simulink model "BrakeActuator"  (Simulink 7.4)
settings: Solver=ode45  StartTime=0.0  StopTime=10.0  RelTol=1e-3
undefined symbols (not defined in the file): Kf, PBmax, TB
settings Model: Creator=alesch  LastModifiedBy=alesch

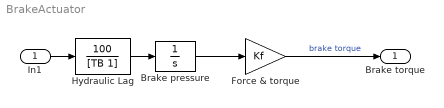
== system BrakeActuator ==
  In1 : Inport  OutDataType=fixdt(1, 16)  OutScaling=2^0
  Brake pressure : Integrator  LimitOutput=on  UpperSaturationLimit=PBmax  LowerSaturationLimit=0
  Force & torque : Gain  Gain=Kf  ParameterDataType=sfix(16)  ParameterScaling=2^0  OutDataType=sfix(16)  OutScaling=2^0  SaturateOnIntegerOverflow=on  OutDataTypeStr=Inherit: Same as input  ParamDataTypeStr=Inherit: Same as input
  "Hydraulic Lag " : TransferFcn  Numerator=[100]  Denominator=[TB 1]
  Brake torque : Outport
  wires:
  Brake pressure/1 -> Force & torque/1
  "Hydraulic Lag "/1 -> Brake pressure/1
  Force & torque/1 -> Brake torque/1  "brake torque"
  In1/1 -> "Hydraulic Lag "/1
